simulink model "RNG_LFSR_4bit_manual"  (R2020a)
settings: Solver=VariableStepAuto  StartTime=0.0  StopTime=15  RelTol=1e-3
PreLoadFcn:
  | fs=1e6
StopFcn:
  | hist(out.simout.data,128)
  | xlabel("Generated Number");
  | ylabel("Number of Occurances");
libraries: simulink_extras x5, hdlsllib x1
settings Model: Creator=ringl  LastModifiedBy=ringl

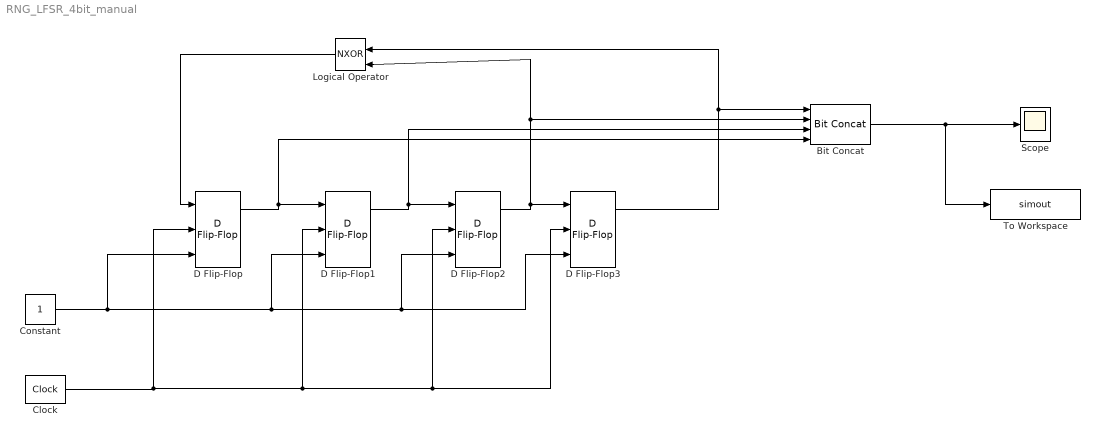
== system RNG_LFSR_4bit_manual ==
  Bit Concat : hdlsllib/Logic and Bit Operations/Bit Concat  numInputs=4
  Clock : simulink_extras/Flip Flops/Clock  period=1
  Constant : Constant
  D Flip-Flop{,1..3} (4 alike) : simulink_extras/Flip Flops/D Flip-Flop
  Logical Operator : Logic  Operator=NXOR  IconShape=distinctive  AllPortsSameDT=off  OutDataTypeStr=boolean
  Scope : Scope
  To Workspace : ToWorkspace  VariableName=simout  SaveFormat=Timeseries  SampleTime=-1
  wires:
  D Flip-Flop/1 -> Bit Concat/4, D Flip-Flop1/1
  D Flip-Flop1/1 -> Bit Concat/3, D Flip-Flop2/1
  D Flip-Flop2/1 -> Logical Operator/2, Bit Concat/2, D Flip-Flop3/1
  D Flip-Flop3/1 -> Bit Concat/1, Logical Operator/1
  Clock/1 -> D Flip-Flop3/2, D Flip-Flop2/2, D Flip-Flop1/2, D Flip-Flop/2
  Logical Operator/1 -> D Flip-Flop/1
  Constant/1 -> D Flip-Flop/3, D Flip-Flop1/3, D Flip-Flop2/3, D Flip-Flop3/3
  Bit Concat/1 -> Scope/1, To Workspace/1
